simulink model "TestSetup"  (R2014b)
settings: Solver=ode45  StartTime=0.0  StopTime=20  RelTol=1e-3
values from neighbouring files (symbols this model uses):
  id = 1    [testSetupRun.m]
  speed = 200    [testSetupRun.m]
  startPos = 400    [testSetupRun.m]
  stopPos = 810    [testSetupRun.m]
undefined symbols (not defined in the file or in its folder): serial
libraries: simulink x6, instrumentlib x3
settings Model: Creator=dan  LastModifiedBy=dan

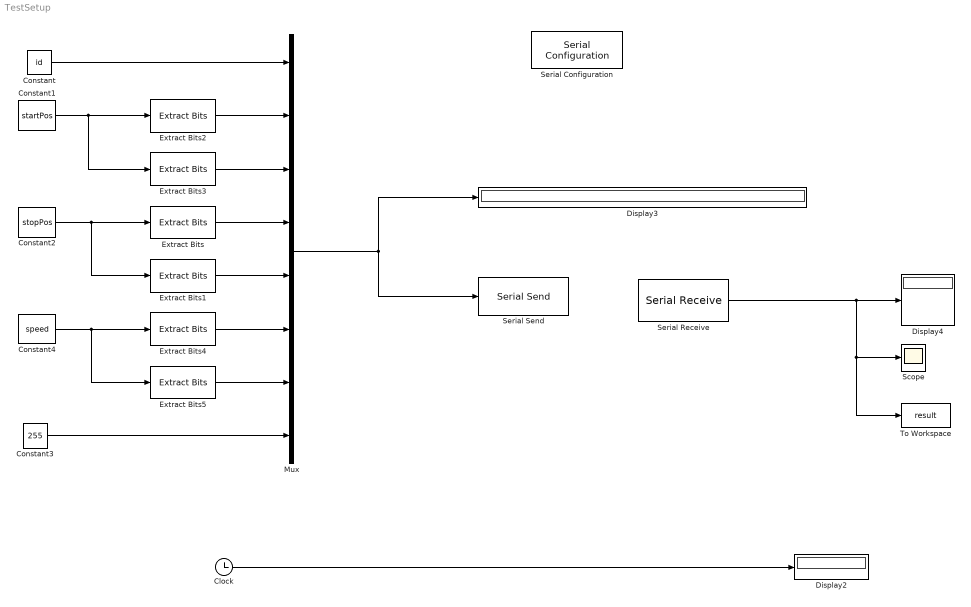
== system TestSetup ==
  Clock : Clock
  Constant : Constant  Value=id  OutDataTypeStr=uint8  SampleTime=1
  Constant1 : Constant  Value=startPos  OutDataTypeStr=uint16  SampleTime=1
  Constant2 : Constant  Value=stopPos  OutDataTypeStr=uint16  SampleTime=1
  Constant3 : Constant  Value=255  OutDataTypeStr=uint8  SampleTime=1
  Constant4 : Constant  Value=speed  OutDataTypeStr=uint16  SampleTime=1
  Display2 : Display
      settings: Format=hex (Stored Integer)
  Display3 : Display
      settings: Format=hex (Stored Integer)
  Display4 : Display
      settings: Format=hex (Stored Integer)
  Extract Bits : simulink/Logic and Bit Operations/Extract Bits  bitsToExtract=Upper half  numBits=8  bitIdxRange=[0 7]  outScalingMode=Treat bit field as an integer
  Extract Bits1 : simulink/Logic and Bit Operations/Extract Bits  bitsToExtract=Lower half  numBits=8  bitIdxRange=[0 7]  outScalingMode=Treat bit field as an integer
  Extract Bits2 : simulink/Logic and Bit Operations/Extract Bits  bitsToExtract=Upper half  numBits=8  bitIdxRange=[0 7]  outScalingMode=Treat bit field as an integer
  Extract Bits3 : simulink/Logic and Bit Operations/Extract Bits  bitsToExtract=Lower half  numBits=8  bitIdxRange=[0 7]  outScalingMode=Treat bit field as an integer
  Extract Bits4 : simulink/Logic and Bit Operations/Extract Bits  bitsToExtract=Upper half  numBits=8  bitIdxRange=[0 7]  outScalingMode=Treat bit field as an integer
  Extract Bits5 : simulink/Logic and Bit Operations/Extract Bits  bitsToExtract=Lower half  numBits=8  bitIdxRange=[0 7]  outScalingMode=Treat bit field as an integer
  Mux : Mux  Inputs=8
  Scope : Scope
      settings: YMin=-30000  YMax=0
  Serial Configuration : instrumentlib/Serial Configuration  Priority=-200000  ComPortMenu=COM4  ComPort=COM4  ObjConstructor=serial('COM4');  BaudRate=115200  DataBits=8  Parity=none  StopBits=1  FlowControl=none  Timeout=0.01  ByteOrder=LittleEndian
  Serial Receive : instrumentlib/Serial Receive  Priority=3  ComPortMenu=COM4  ComPort=COM4  ObjConstructor=serial('COM4');  Terminator=<none>  DataSize=3  DataType=int16  EnableBlockingMode=on  ActionDataUnavailable=Output custom value  CustomValue=0  SampleTime=0.01
  Serial Send : instrumentlib/Serial Send  Priority=2  ComPortMenu=COM4  ComPort=COM4  ObjConstructor=serial('COM4');  Terminator=<none>  EnableBlockingMode=on
  To Workspace : ToWorkspace  VariableName=result  SampleTime=-1
      settings: Save2DSignal=2-D array (concatenate along first dimension)
  wires:
  Clock/1 -> Display2/1
  Constant/1 -> Mux/1
  Extract Bits/1 -> Mux/4
  Constant2/1 -> Extract Bits1/1, Extract Bits/1
  Extract Bits1/1 -> Mux/5
  Extract Bits3/1 -> Mux/3
  Extract Bits2/1 -> Mux/2
  Constant1/1 -> Extract Bits3/1, Extract Bits2/1
  Mux/1 -> Display3/1, Serial Send/1
  Serial Receive/1 -> To Workspace/1, Scope/1, Display4/1
  Constant3/1 -> Mux/8
  Extract Bits4/1 -> Mux/6
  Constant4/1 -> Extract Bits5/1, Extract Bits4/1
  Extract Bits5/1 -> Mux/7
